simulink model "Model_mnogocanal_system_svyazi_s_chast_razd_canalov"  (R2023b)
settings: Solver=VariableStepAuto  StartTime=0.0  StopTime=0.000005  RelTol=1e-3
libraries: simulink_extras x13, dspfdesign x9, simulink x2
settings Model: Creator=User  LastModifiedBy=User

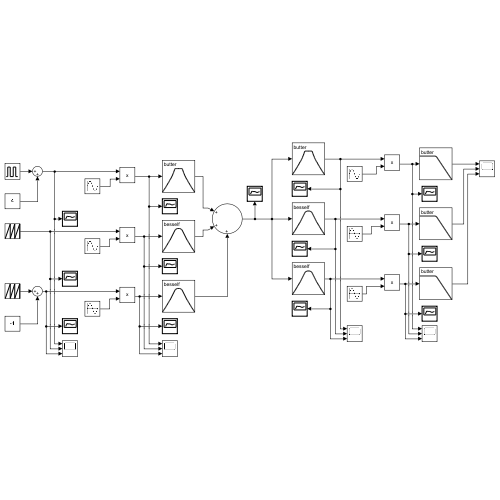
[thumbnail: Simulink's stored preview of the top-level diagram]
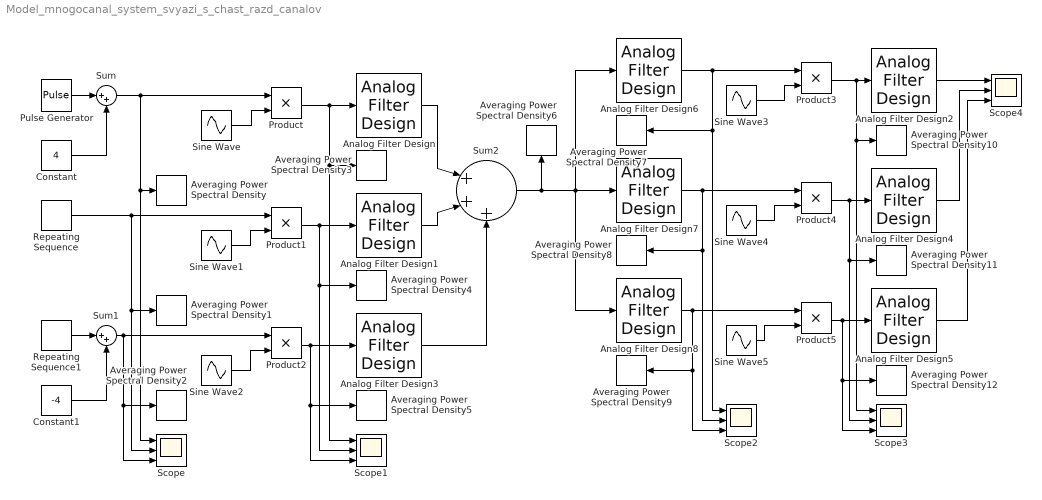
== system Model_mnogocanal_system_svyazi_s_chast_razd_canalov ==
  Analog Filter Design : dspfdesign/Analog Filter Design  method=Butterworth  filttype=Bandpass  N=8  Wlo=30  Whi=80  Rp=2  Rs=40
  Analog Filter Design{1,3,7..8} (4 alike) : dspfdesign/Analog Filter Design  method=Bessel  filttype=Bandpass  N=8  Wlo=30  Whi=80  Rp=2  Rs=40
  Analog Filter Design2 : dspfdesign/Analog Filter Design  method=Butterworth  filttype=Lowpass  N=8  Wlo=30  Whi=80  Rp=2  Rs=40
  Analog Filter Design4 : dspfdesign/Analog Filter Design  method=Butterworth  filttype=Lowpass  N=8  Wlo=30  Whi=80  Rp=2  Rs=40
  Analog Filter Design5 : dspfdesign/Analog Filter Design  method=Butterworth  filttype=Lowpass  N=8  Wlo=30  Whi=80  Rp=2  Rs=40
  Analog Filter Design6 : dspfdesign/Analog Filter Design  method=Butterworth  filttype=Bandpass  N=8  Wlo=30  Whi=80  Rp=2  Rs=40
  Averaging Power Spectral Density{,1..12} (13 alike) : simulink_extras/Additional Sinks/Averaging Power Spectral Density  npts=128  fftpts=512  HowOften=64  sampleT=0.000005
  Constant : Constant  Value=4
  Constant1 : Constant  Value=-4
  Product{,1..5} (6 alike) : Product
  Pulse Generator : DiscretePulseGenerator  PulseType=Time based  Amplitude=3  Period=0.4*10^(-6)  PulseWidth=50
  Repeating Sequence : simulink/Sources/Repeating Sequence  rep_seq_t=[0 2*10^(-6)]  rep_seq_y=[0 3]
  Repeating Sequence1 : simulink/Sources/Repeating Sequence  rep_seq_t=[0 0.3*10^(-6)]  rep_seq_y=[0 4.5]
  Scope{,1..4} (5 alike) : Scope  NumInputPorts=3
  Sine Wave : Sin  Amplitude=3  Frequency=10*10^6  SampleTime=0
  Sine Wave1 : Sin  Amplitude=3  Frequency=15*10^6  SampleTime=0
  Sine Wave2 : Sin  Amplitude=3  Frequency=21*10^6  SampleTime=0
  Sine Wave3 : Sin  Amplitude=3  Frequency=10*10^6  SampleTime=0
  Sine Wave4 : Sin  Amplitude=3  Frequency=15*10^6  SampleTime=0
  Sine Wave5 : Sin  Amplitude=3  Frequency=21*10^6  SampleTime=0
  Sum : Sum  Inputs=|++
  Sum1 : Sum  Inputs=|++
  Sum2 : Sum  Inputs=|+++
  wires:
  Pulse Generator/1 -> Sum/1
  Constant/1 -> Sum/2
  Repeating Sequence1/1 -> Sum1/1
  Constant1/1 -> Sum1/2
  Analog Filter Design2/1 -> Scope4/1
  Analog Filter Design4/1 -> Scope4/2
  Analog Filter Design5/1 -> Scope4/3
  Product5/1 -> Averaging Power Spectral Density12/1, Scope3/3, Analog Filter Design5/1
  Product3/1 -> Averaging Power Spectral Density10/1, Scope3/1, Analog Filter Design2/1
  Product4/1 -> Averaging Power Spectral Density11/1, Scope3/2, Analog Filter Design4/1
  Sine Wave4/1 -> Product4/2
  Sine Wave3/1 -> Product3/2
  Sine Wave5/1 -> Product5/2
  Sum2/1 -> Analog Filter Design8/1, Analog Filter Design6/1, Analog Filter Design7/1, Averaging Power Spectral Density6/1
  Sine Wave1/1 -> Product1/2
  Sine Wave2/1 -> Product2/2
  Sine Wave/1 -> Product/2
  Sum1/1 -> Product2/1, Averaging Power Spectral Density2/1, Scope/3
  Repeating Sequence/1 -> Product1/1, Averaging Power Spectral Density1/1, Scope/2
  Sum/1 -> Product/1, Averaging Power Spectral Density/1, Scope/1
  Product/1 -> Analog Filter Design/1, Averaging Power Spectral Density3/1, Scope1/1
  Product1/1 -> Analog Filter Design1/1, Averaging Power Spectral Density4/1, Scope1/2
  Product2/1 -> Analog Filter Design3/1, Averaging Power Spectral Density5/1, Scope1/3
  Analog Filter Design/1 -> Sum2/1
  Analog Filter Design1/1 -> Sum2/2
  Analog Filter Design3/1 -> Sum2/3
  Analog Filter Design7/1 -> Averaging Power Spectral Density8/1, Scope2/2, Product4/1
  Analog Filter Design6/1 -> Averaging Power Spectral Density7/1, Scope2/1, Product3/1
  Analog Filter Design8/1 -> Averaging Power Spectral Density9/1, Scope2/3, Product5/1
